simulink model "nms_model"  (R2020a)
settings: Solver=ode15s  StartTime=0.0  StopTime=2.6  MaxStep=.01  RelTol=1e-4  AbsTol=1e-6  EnableMultiTasking=on
values from neighbouring files (symbols this model uses):
  dt_visual = -1    [NMScontrol.m]    (also in runmodel.m = 0.001)
  g = params.g    [NMPCcostFunction.m]    (also in dynamicsNMPC.m = 9.81)
  m = parametersOpt(1)    [CGBgreybox.m]    (also in NMPCcostFunction.m = params.m)
undefined symbols (not defined in the file or in its folder): hatLeftHipToCenterDistWidth, initialTargetAngle, LongDelay, LongLoopDelay, LPreStimBFSHinit, LPreStimGASinit, LPreStimGLUinit, LPreStimHABinit, LPreStimHADinit, LPreStimHAMinit, LPreStimHFLinit, LPreStimRFinit, LPreStimSOLinit, LPreStimTAinit, LPreStimVASinit, LTargetAngleInit, LTargetAngleRInit, MidDelay, RPreStimBFSHinit, RPreStimGASinit, RPreStimGLUinit, RPreStimHABinit, RPreStimHADinit, RPreStimHAMinit, RPreStimHFLinit, RPreStimRFinit, RPreStimSOLinit, RPreStimTAinit, RPreStimVASinit, RTargetAngleInit, RTargetAngleRInit, ShortDelay, termination_height, thetaHATref, X, Y, Z
libraries: NeuroMuscularLibrary x107, nesl_utility x25, sm_lib x16, simulink x3
(part 3 of 3)

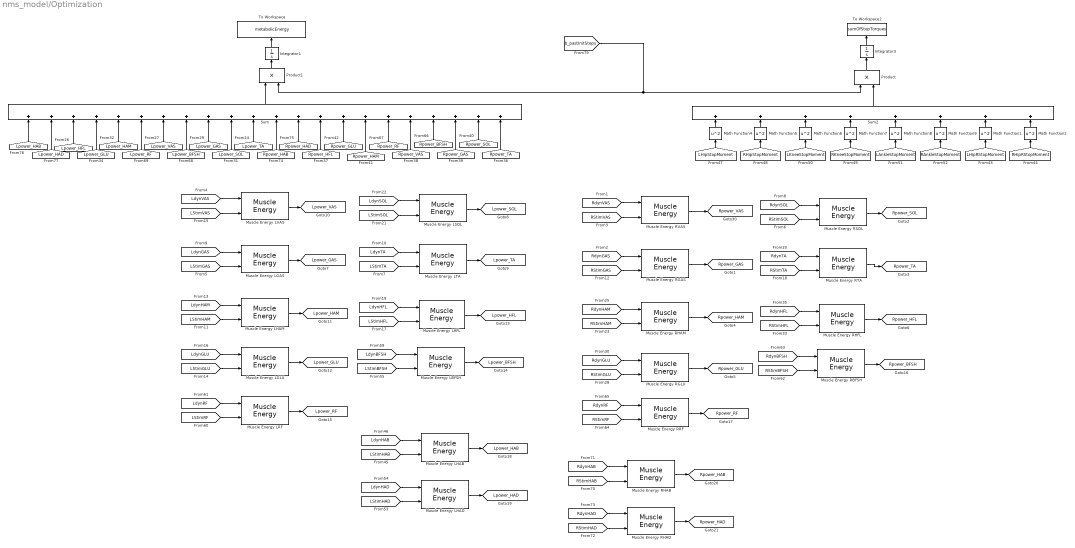
== system nms_model/Optimization ==
  Integrator1 : Integrator
  Integrator3 : Integrator
  Math Function{1..2,4..9} (8 alike) : Math  Operator=square  SignedPower=on  SaturateOnIntegerOverflow=on
  Muscle Energy LBFSH : NeuroMuscularLibrary/Muscle Energy  lopt=loptBFSH  FT=FT_BFSH  Fmax=FmaxBFSH  vmax=vmaxBFSH
  Muscle Energy LGAS : NeuroMuscularLibrary/Muscle Energy  lopt=loptGAS  FT=FT_GAS  Fmax=FmaxGAS  vmax=vmaxGAS
  Muscle Energy LGLU : NeuroMuscularLibrary/Muscle Energy  lopt=loptGLU  FT=FT_GLU  Fmax=FmaxGLU  vmax=vmaxGLU
  Muscle Energy LHAB : NeuroMuscularLibrary/Muscle Energy  lopt=loptHAB  FT=FT_HAB  Fmax=FmaxHAB  vmax=vmaxHAB
  Muscle Energy LHAD : NeuroMuscularLibrary/Muscle Energy  lopt=loptHAD  FT=FT_HAD  Fmax=FmaxHAD  vmax=vmaxHAD
  Muscle Energy LHAM : NeuroMuscularLibrary/Muscle Energy  lopt=loptHAM  FT=FT_HAM  Fmax=FmaxHAM  vmax=vmaxHAM
  Muscle Energy LHFL : NeuroMuscularLibrary/Muscle Energy  lopt=loptHFL  FT=FT_HFL  Fmax=FmaxHFL  vmax=vmaxHFL
  Muscle Energy LRF : NeuroMuscularLibrary/Muscle Energy  lopt=loptRF  FT=FT_RF  Fmax=FmaxRF  vmax=vmaxRF
  Muscle Energy LSOL : NeuroMuscularLibrary/Muscle Energy  lopt=loptSOL  FT=FT_SOL  Fmax=FmaxSOL  vmax=vmaxSOL
  Muscle Energy LTA : NeuroMuscularLibrary/Muscle Energy  lopt=loptTA  FT=FT_TA  Fmax=FmaxTA  vmax=vmaxTA
  Muscle Energy LVAS : NeuroMuscularLibrary/Muscle Energy  lopt=loptVAS  FT=FT_VAS  Fmax=FmaxVAS  vmax=vmaxVAS
  Muscle Energy RBFSH : NeuroMuscularLibrary/Muscle Energy  lopt=loptBFSH  FT=FT_BFSH  Fmax=FmaxBFSH  vmax=vmaxBFSH
  Muscle Energy RGAS : NeuroMuscularLibrary/Muscle Energy  lopt=loptGAS  FT=FT_GAS  Fmax=FmaxGAS  vmax=vmaxGAS
  Muscle Energy RGLU : NeuroMuscularLibrary/Muscle Energy  lopt=loptGLU  FT=FT_GLU  Fmax=FmaxGLU  vmax=vmaxGLU
  Muscle Energy RHAB : NeuroMuscularLibrary/Muscle Energy  lopt=loptHAB  FT=FT_HAB  Fmax=FmaxHAB  vmax=vmaxHAB
  Muscle Energy RHAD : NeuroMuscularLibrary/Muscle Energy  lopt=loptHAD  FT=FT_HAD  Fmax=FmaxHAD  vmax=vmaxHAD
  Muscle Energy RHAM : NeuroMuscularLibrary/Muscle Energy  lopt=loptHAM  FT=FT_HAM  Fmax=FmaxHAM  vmax=vmaxHAM
  Muscle Energy RHFL : NeuroMuscularLibrary/Muscle Energy  lopt=loptHFL  FT=FT_HFL  Fmax=FmaxHFL  vmax=vmaxHFL
  Muscle Energy RRF : NeuroMuscularLibrary/Muscle Energy  lopt=loptRF  FT=FT_RF  Fmax=FmaxRF  vmax=vmaxRF
  Muscle Energy RSOL : NeuroMuscularLibrary/Muscle Energy  lopt=loptSOL  FT=FT_SOL  Fmax=FmaxSOL  vmax=vmaxSOL
  Muscle Energy RTA : NeuroMuscularLibrary/Muscle Energy  lopt=loptTA  FT=FT_TA  Fmax=FmaxTA  vmax=vmaxTA
  Muscle Energy RVAS : NeuroMuscularLibrary/Muscle Energy  lopt=loptVAS  FT=FT_VAS  Fmax=FmaxVAS  vmax=vmaxVAS
  Product : Product
  Product1 : Product
  Sum : Sum  Inputs=++++++++++++++++++++++
  Sum2 : Sum  Inputs=++++++++
  To Workspace : ToWorkspace  VariableName=metabolicEnergy  SampleTime=-1
      settings: MaxDataPoints=1
  To Workspace2 : ToWorkspace  VariableName=sumOfStopTorques  SampleTime=-1
      settings: MaxDataPoints=1
  tag scope: Lpower_BFSH=global, Lpower_GAS=global, Lpower_GLU=global, Lpower_HAB=global, Lpower_HAD=global, Lpower_HAM=global, Lpower_HFL=global, Lpower_RF=global, Lpower_SOL=global, Lpower_TA=global, Lpower_VAS=global, Rpower_BFSH=global, Rpower_GAS=global, Rpower_GLU=global, Rpower_HAB=global, Rpower_HAD=global, Rpower_HAM=global, Rpower_HFL=global, Rpower_RF=global, Rpower_SOL=global, Rpower_TA=global, Rpower_VAS=global
  wires:
  [RdynSOL] -> Muscle Energy RSOL/1
  [RStimSOL] -> Muscle Energy RSOL/2
  [RStimVAS] -> Muscle Energy RVAS/2
  [RStimGAS] -> Muscle Energy RGAS/2
  Muscle Energy RVAS/1 -> [Rpower_VAS]
  Muscle Energy RGAS/1 -> [Rpower_GAS]
  Muscle Energy RSOL/1 -> [Rpower_SOL]
  Muscle Energy RTA/1 -> [Rpower_TA]
  [RdynTA] -> Muscle Energy RTA/1
  [RStimTA] -> Muscle Energy RTA/2
  [RdynHAM] -> Muscle Energy RHAM/1
  [RStimHAM] -> Muscle Energy RHAM/2
  [RdynGLU] -> Muscle Energy RGLU/1
  [RStimGLU] -> Muscle Energy RGLU/2
  [RdynHFL] -> Muscle Energy RHFL/1
  [RStimHFL] -> Muscle Energy RHFL/2
  Muscle Energy RHAM/1 -> [Rpower_HAM]
  Muscle Energy RGLU/1 -> [Rpower_GLU]
  Muscle Energy RHFL/1 -> [Rpower_HFL]
  [Lpower_HAB] -> Sum/1
  [Lpower_VAS] -> Sum/7
  [Lpower_RF] -> Sum/6
  [Lpower_HAM] -> Sum/5
  [Lpower_GLU] -> Sum/4
  [Lpower_HFL] -> Sum/3
  [Lpower_HAD] -> Sum/2
  [RdynGAS] -> Muscle Energy RGAS/1
  [RdynVAS] -> Muscle Energy RVAS/1
  [LdynSOL] -> Muscle Energy LSOL/1
  [LStimSOL] -> Muscle Energy LSOL/2
  [LStimVAS] -> Muscle Energy LVAS/2
  [LStimGAS] -> Muscle Energy LGAS/2
  Muscle Energy LVAS/1 -> [Lpower_VAS]
  Muscle Energy LGAS/1 -> [Lpower_GAS]
  Muscle Energy LSOL/1 -> [Lpower_SOL]
  Muscle Energy LTA/1 -> [Lpower_TA]
  [LdynTA] -> Muscle Energy LTA/1
  [LStimTA] -> Muscle Energy LTA/2
  [LdynHAM] -> Muscle Energy LHAM/1
  [LStimHAM] -> Muscle Energy LHAM/2
  [LdynGLU] -> Muscle Energy LGLU/1
  [LStimGLU] -> Muscle Energy LGLU/2
  [LdynHFL] -> Muscle Energy LHFL/1
  [LStimHFL] -> Muscle Energy LHFL/2
  Muscle Energy LHAM/1 -> [Lpower_HAM]
  Muscle Energy LGLU/1 -> [Lpower_GLU]
  Muscle Energy LHFL/1 -> [Lpower_HFL]
  [LdynGAS] -> Muscle Energy LGAS/1
  [LdynVAS] -> Muscle Energy LVAS/1
  [Lpower_SOL] -> Sum/10
  [Rpower_HAM] -> Sum/16
  [Rpower_GLU] -> Sum/15
  [Rpower_HFL] -> Sum/14
  [Rpower_HAD] -> Sum/13
  [Rpower_HAB] -> Sum/12
  [Lpower_TA] -> Sum/11
  Integrator1/1 -> To Workspace/1
  Sum/1 -> Product1/1
  Integrator3/1 -> To Workspace2/1
  Math Function4/1 -> Sum2/1
  [LHipStopMoment] -> Math Function4/1
  Math Function5/1 -> Sum2/2
  [RHipStopMoment] -> Math Function5/1
  Math Function6/1 -> Sum2/3
  Math Function7/1 -> Sum2/4
  [LKneeStopMoment] -> Math Function6/1
  [RKneeStopMoment] -> Math Function7/1
  [LAnkleStopMoment] -> Math Function8/1
  Math Function8/1 -> Sum2/5
  [RAnkleStopMoment] -> Math Function9/1
  Math Function9/1 -> Sum2/6
  Product/1 -> Integrator3/1
  Sum2/1 -> Product/2
  Product1/1 -> Integrator1/1
  Muscle Energy LBFSH/1 -> [Lpower_BFSH]
  [LStimBFSH] -> Muscle Energy LBFSH/2
  [LdynBFSH] -> Muscle Energy LBFSH/1
  [LdynRF] -> Muscle Energy LRF/1
  [LStimRF] -> Muscle Energy LRF/2
  Muscle Energy LRF/1 -> [Lpower_RF]
  Muscle Energy RRF/1 -> [Rpower_RF]
  [RdynRF] -> Muscle Energy RRF/1
  Muscle Energy RBFSH/1 -> [Rpower_BFSH]
  [RStimRF] -> Muscle Energy RRF/2
  [RStimBFSH] -> Muscle Energy RBFSH/2
  [RdynBFSH] -> Muscle Energy RBFSH/1
  [Lpower_BFSH] -> Sum/8
  [Lpower_GAS] -> Sum/9
  [Rpower_VAS] -> Sum/18
  [Rpower_RF] -> Sum/17
  Math Function1/1 -> Sum2/7
  [LHipRStopMoment] -> Math Function1/1
  [RHipRStopMoment] -> Math Function2/1
  Muscle Energy LHAB/1 -> [Lpower_HAB]
  [LStimHAB] -> Muscle Energy LHAB/2
  [LdynHAB] -> Muscle Energy LHAB/1
  [LdynHAD] -> Muscle Energy LHAD/1
  [LStimHAD] -> Muscle Energy LHAD/2
  Muscle Energy LHAD/1 -> [Lpower_HAD]
  Muscle Energy RHAD/1 -> [Rpower_HAD]
  [RStimHAD] -> Muscle Energy RHAD/2
  [RdynHAD] -> Muscle Energy RHAD/1
  [RdynHAB] -> Muscle Energy RHAB/1
  [RStimHAB] -> Muscle Energy RHAB/2
  Muscle Energy RHAB/1 -> [Rpower_HAB]
  [Rpower_TA] -> Sum/22
  [Rpower_SOL] -> Sum/21
  [Rpower_GAS] -> Sum/20
  [Rpower_BFSH] -> Sum/19
  Math Function2/1 -> Sum2/8
  [b_pastInitSteps] -> Product/1, Product1/2

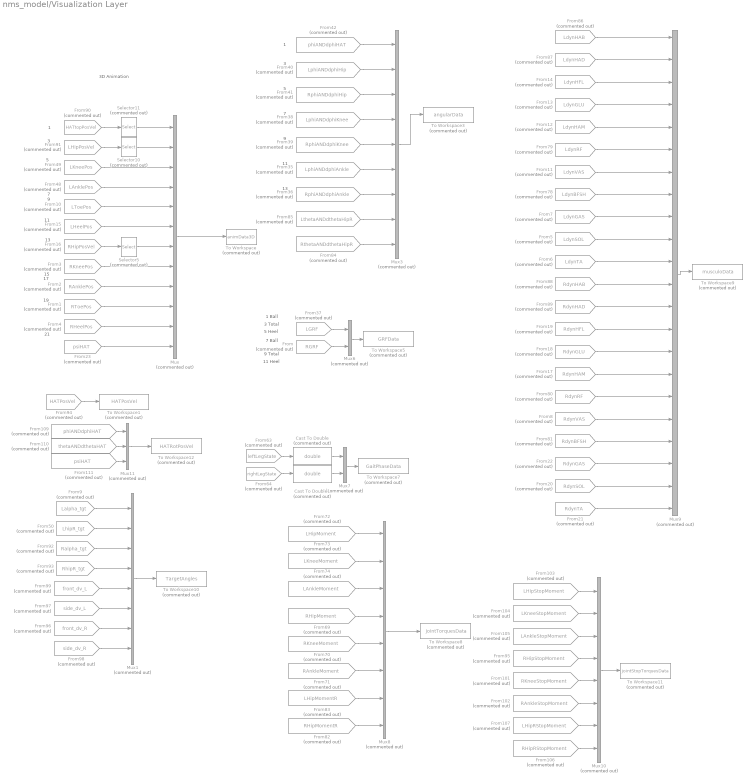
== system nms_model/Visualization Layer ==
  note: 21
  note: 19
  note: 17
  note: 15
  note: 13
  note: 11
  note: 9
  note: 7
  note: 5
  note: 3
  note: 1
  note: 3D Animation
  note: 1
  note: 13
  note: 3
  note: 5
  note: 7
  note: 9
  note: 11
  note: 9 Total
  note: 1 Ball
  note: 5 Heel
  note: 11 Heel
  note: 3 Total
  note: 7 Ball
  Cast To Double : DataTypeConversion  Commented=on  OutDataTypeStr=double
  Cast To Double1 : DataTypeConversion  Commented=on  OutDataTypeStr=double
  From : From  Commented=on  GotoTag=RGRF  TagVisibility=global
  From1 : From  Commented=on  GotoTag=RToePos  TagVisibility=global
      settings: CloseFcn=tagdialog Close
  From10 : From  Commented=on  GotoTag=LToePos  TagVisibility=global
      settings: CloseFcn=tagdialog Close
  From101 : From  Commented=on  GotoTag=RKneeStopMoment  TagVisibility=global
  From102 : From  Commented=on  GotoTag=RAnkleStopMoment  TagVisibility=global
  From103 : From  Commented=on  GotoTag=LHipStopMoment  TagVisibility=global
  From104 : From  Commented=on  GotoTag=LKneeStopMoment  TagVisibility=global
  From105 : From  Commented=on  GotoTag=LAnkleStopMoment  TagVisibility=global
  From106 : From  Commented=on  GotoTag=RHipRStopMoment  TagVisibility=global
  From107 : From  Commented=on  GotoTag=LHipRStopMoment  TagVisibility=global
  From109 : From  Commented=on  GotoTag=phiANDdphiHAT  TagVisibility=global
  From11 : From  Commented=on  GotoTag=LdynVAS  TagVisibility=global
  From110 : From  Commented=on  GotoTag=thetaANDdthetaHAT  TagVisibility=global
  From111 : From  Commented=on  GotoTag=psiHAT  TagVisibility=global
  From12 : From  Commented=on  GotoTag=LdynHAM  TagVisibility=global
  From13 : From  Commented=on  GotoTag=LdynGLU  TagVisibility=global
  From14 : From  Commented=on  GotoTag=LdynHFL  TagVisibility=global
  From15 : From  Commented=on  GotoTag=LHeelPos  TagVisibility=global
      settings: CloseFcn=tagdialog Close
  From16 : From  Commented=on  GotoTag=RHipPosVel  TagVisibility=global
  From17 : From  Commented=on  GotoTag=RdynHAM  TagVisibility=global
  From18 : From  Commented=on  GotoTag=RdynGLU  TagVisibility=global
  From19 : From  Commented=on  GotoTag=RdynHFL  TagVisibility=global
  From2 : From  Commented=on  GotoTag=RAnklePos  TagVisibility=global
      settings: CloseFcn=tagdialog Close
  From20 : From  Commented=on  GotoTag=RdynSOL  TagVisibility=global
  From21 : From  Commented=on  GotoTag=RdynTA  TagVisibility=global
  From22 : From  Commented=on  GotoTag=RdynGAS  TagVisibility=global
  From23 : From  Commented=on  GotoTag=psiHAT  TagVisibility=global
  From3 : From  Commented=on  GotoTag=RKneePos  TagVisibility=global
      settings: CloseFcn=tagdialog Close
  From35 : From  Commented=on  GotoTag=LphiANDdphiAnkle  TagVisibility=global
  From36 : From  Commented=on  GotoTag=RphiANDdphiAnkle  TagVisibility=global
  From37 : From  Commented=on  GotoTag=LGRF  TagVisibility=global
  From38 : From  Commented=on  GotoTag=LphiANDdphiKnee  TagVisibility=global
  From39 : From  Commented=on  GotoTag=RphiANDdphiKnee  TagVisibility=global
  From4 : From  Commented=on  GotoTag=RHeelPos  TagVisibility=global
      settings: CloseFcn=tagdialog Close
  From40 : From  Commented=on  GotoTag=LphiANDdphiHip  TagVisibility=global
  From41 : From  Commented=on  GotoTag=RphiANDdphiHip  TagVisibility=global
  From42 : From  Commented=on  GotoTag=phiANDdphiHAT  TagVisibility=global
  From48 : From  Commented=on  GotoTag=LAnklePos  TagVisibility=global
      settings: CloseFcn=tagdialog Close
  From49 : From  Commented=on  GotoTag=LKneePos  TagVisibility=global
      settings: CloseFcn=tagdialog Close
  From5 : From  Commented=on  GotoTag=LdynSOL  TagVisibility=global
  From50 : From  Commented=on  GotoTag=LhipR_tgt  TagVisibility=global
  From6 : From  Commented=on  GotoTag=LdynTA  TagVisibility=global
  From63 : From  Commented=on  GotoTag=leftLegState  TagVisibility=global
  From64 : From  Commented=on  GotoTag=rightLegState  TagVisibility=global
  From69 : From  Commented=on  GotoTag=RHipMoment  TagVisibility=global
  From7 : From  Commented=on  GotoTag=LdynGAS  TagVisibility=global
  From70 : From  Commented=on  GotoTag=RKneeMoment  TagVisibility=global
  From71 : From  Commented=on  GotoTag=RAnkleMoment  TagVisibility=global
  From72 : From  Commented=on  GotoTag=LHipMoment  TagVisibility=global
  From73 : From  Commented=on  GotoTag=LKneeMoment  TagVisibility=global
  From74 : From  Commented=on  GotoTag=LAnkleMoment  TagVisibility=global
  From78 : From  Commented=on  GotoTag=LdynBFSH  TagVisibility=global
  From79 : From  Commented=on  GotoTag=LdynRF  TagVisibility=global
  From8 : From  Commented=on  GotoTag=RdynVAS  TagVisibility=global
  From80 : From  Commented=on  GotoTag=RdynRF  TagVisibility=global
  From81 : From  Commented=on  GotoTag=RdynBFSH  TagVisibility=global
  From82 : From  Commented=on  GotoTag=RHipMomentR  TagVisibility=global
  From83 : From  Commented=on  GotoTag=LHipMomentR  TagVisibility=global
  From84 : From  Commented=on  GotoTag=RthetaANDdthetaHipR  TagVisibility=global
  From85 : From  Commented=on  GotoTag=LthetaANDdthetaHipR  TagVisibility=global
  From86 : From  Commented=on  GotoTag=LdynHAB  TagVisibility=global
  From87 : From  Commented=on  GotoTag=LdynHAD  TagVisibility=global
  From88 : From  Commented=on  GotoTag=RdynHAB  TagVisibility=global
  From89 : From  Commented=on  GotoTag=RdynHAD  TagVisibility=global
  From9 : From  Commented=on  GotoTag=Lalpha_tgt  TagVisibility=global
  From90 : From  Commented=on  GotoTag=HATtopPosVel  TagVisibility=global
  From91 : From  Commented=on  GotoTag=LHipPosVel  TagVisibility=global
  From92 : From  Commented=on  GotoTag=Ralpha_tgt  TagVisibility=global
  From93 : From  Commented=on  GotoTag=RhipR_tgt  TagVisibility=global
  From94 : From  Commented=on  GotoTag=HATPosVel  TagVisibility=global
  From95 : From  Commented=on  GotoTag=RHipStopMoment  TagVisibility=global
  From96 : From  Commented=on  GotoTag=front_dv_R  TagVisibility=global
      settings: CloseFcn=tagdialog Close
  From97 : From  Commented=on  GotoTag=side_dv_L  TagVisibility=global
      settings: CloseFcn=tagdialog Close
  From98 : From  Commented=on  GotoTag=side_dv_R  TagVisibility=global
      settings: CloseFcn=tagdialog Close
  From99 : From  Commented=on  GotoTag=front_dv_L  TagVisibility=global
      settings: CloseFcn=tagdialog Close
  Mux : Mux  Commented=on  Inputs=12
  Mux1 : Mux  Commented=on  Inputs=8
  Mux10 : Mux  Commented=on  Inputs=8
  Mux11 : Mux  Commented=on  Inputs=3
  Mux3 : Mux  Commented=on  Inputs=9
  Mux6 : Mux  Commented=on  Inputs=2
  Mux7 : Mux  Commented=on  Inputs=2
  Mux8 : Mux  Commented=on  Inputs=8
  Mux9 : Mux  Commented=on  Inputs=22
  Selector10 : Selector  Commented=on  InputPortWidth=6  IndexOptions=Index vector (dialog)  Indices=[1 2 3]  OutputSizes=1
  Selector11 : Selector  Commented=on  InputPortWidth=6  IndexOptions=Index vector (dialog)  Indices=[1 2 3]  OutputSizes=1
  Selector5 : Selector  Commented=on  InputPortWidth=6  IndexOptions=Index vector (dialog)  Indices=[1 2 3]  OutputSizes=1
  To Workspace : ToWorkspace  Commented=on  VariableName=animData3D  SaveFormat=Structure With Time  SampleTime=-1
  To Workspace1 : ToWorkspace  Commented=on  VariableName=HATPosVel  SaveFormat=Structure With Time  SampleTime=dt_visual
  To Workspace10 : ToWorkspace  Commented=on  VariableName=TargetAngles  SaveFormat=Structure With Time  SampleTime=dt_visual
  To Workspace11 : ToWorkspace  Commented=on  VariableName=jointStopTorquesData  SaveFormat=Structure With Time  SampleTime=dt_visual
  To Workspace12 : ToWorkspace  Commented=on  VariableName=HATRotPosVel  SaveFormat=Structure With Time  SampleTime=dt_visual
  To Workspace3 : ToWorkspace  Commented=on  VariableName=angularData  SaveFormat=Structure With Time  SampleTime=dt_visual
  To Workspace5 : ToWorkspace  Commented=on  VariableName=GRFData  SaveFormat=Structure With Time  SampleTime=dt_visual
  To Workspace7 : ToWorkspace  Commented=on  VariableName=GaitPhaseData  SaveFormat=Structure With Time  SampleTime=dt_visual
  To Workspace8 : ToWorkspace  Commented=on  VariableName=jointTorquesData  SaveFormat=Structure With Time  SampleTime=dt_visual
  To Workspace9 : ToWorkspace  Commented=on  VariableName=musculoData  SaveFormat=Structure With Time  SampleTime=dt_visual
  wires:
  From16/1 -> Selector5/1
  From90/1 -> Selector11/1
  From91/1 -> Selector10/1
  Selector11/1 -> Mux/1
  From2/1 -> Mux/9
  From3/1 -> Mux/8
  Selector5/1 -> Mux/7
  From15/1 -> Mux/6
  From10/1 -> Mux/5
  From48/1 -> Mux/4
  From49/1 -> Mux/3
  Selector10/1 -> Mux/2
  Mux/1 -> To Workspace/1
  From4/1 -> Mux/11
  From1/1 -> Mux/10
  From36/1 -> Mux3/7
  Mux6/1 -> To Workspace5/1
  From/1 -> Mux6/2
  From42/1 -> Mux3/1
  Mux3/1 -> To Workspace3/1
  From35/1 -> Mux3/6
  From38/1 -> Mux3/4
  From37/1 -> Mux6/1
  From40/1 -> Mux3/2
  From39/1 -> Mux3/5
  From41/1 -> Mux3/3
  From64/1 -> Cast To Double1/1
  Mux7/1 -> To Workspace7/1
  From63/1 -> Cast To Double/1
  Mux8/1 -> To Workspace8/1
  From72/1 -> Mux8/1
  From73/1 -> Mux8/2
  From74/1 -> Mux8/3
  From69/1 -> Mux8/4
  From70/1 -> Mux8/5
  From71/1 -> Mux8/6
  Mux9/1 -> To Workspace9/1
  From17/1 -> Mux9/16
  From14/1 -> Mux9/3
  From18/1 -> Mux9/15
  From8/1 -> Mux9/18
  From78/1 -> Mux9/8
  From22/1 -> Mux9/20
  From81/1 -> Mux9/19
  From11/1 -> Mux9/7
  From7/1 -> Mux9/9
  From5/1 -> Mux9/10
  From79/1 -> Mux9/6
  From12/1 -> Mux9/5
  From13/1 -> Mux9/4
  From6/1 -> Mux9/11
  From80/1 -> Mux9/17
  From19/1 -> Mux9/14
  From20/1 -> Mux9/21
  From21/1 -> Mux9/22
  From83/1 -> Mux8/7
  From82/1 -> Mux8/8
  From85/1 -> Mux3/8
  From84/1 -> Mux3/9
  From88/1 -> Mux9/12
  From89/1 -> Mux9/13
  From86/1 -> Mux9/1
  From87/1 -> Mux9/2
  From94/1 -> To Workspace1/1
  From99/1 -> Mux1/5
  From92/1 -> Mux1/3
  From93/1 -> Mux1/4
  Mux1/1 -> To Workspace10/1
  From96/1 -> Mux1/7
  From50/1 -> Mux1/2
  From98/1 -> Mux1/8
  From97/1 -> Mux1/6
  From9/1 -> Mux1/1
  From102/1 -> Mux10/6
  From95/1 -> Mux10/4
  From104/1 -> Mux10/2
  Mux10/1 -> To Workspace11/1
  From103/1 -> Mux10/1
  From101/1 -> Mux10/5
  From105/1 -> Mux10/3
  From107/1 -> Mux10/7
  From106/1 -> Mux10/8
  Mux11/1 -> To Workspace12/1
  From110/1 -> Mux11/2
  From111/1 -> Mux11/3
  From109/1 -> Mux11/1
  From23/1 -> Mux/12
  Cast To Double/1 -> Mux7/1
  Cast To Double1/1 -> Mux7/2

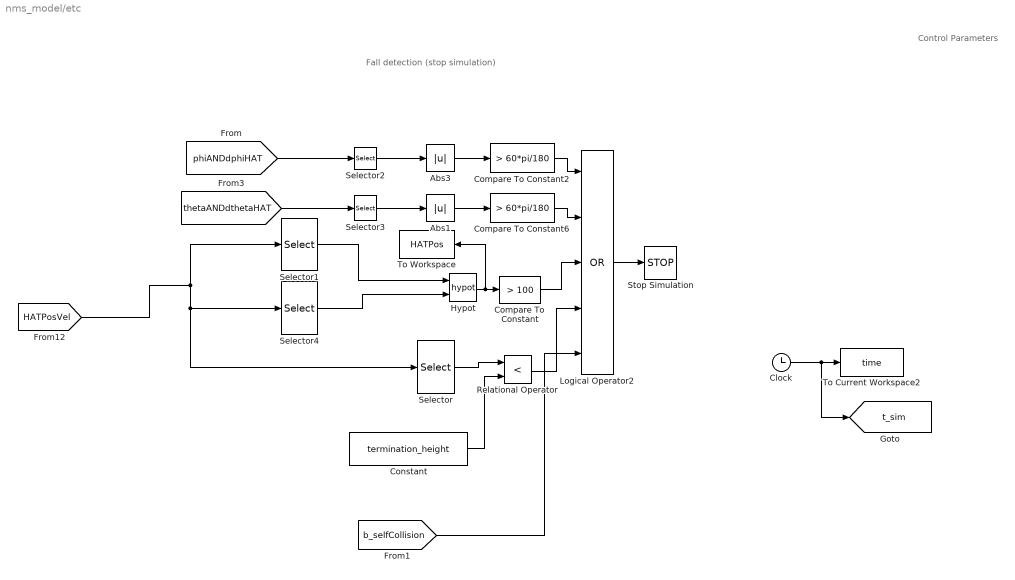
== system nms_model/etc ==
  note: Fall detection
      | (stop simulation)
  note: Control Parameters
  Abs1 : Abs
  Abs3 : Abs
  Clock : Clock
  Compare To Constant : simulink/Logic and Bit Operations/Compare To Constant  relop=>  const=100  OutDataTypeStr=boolean
  Compare To Constant2 : simulink/Logic and Bit Operations/Compare To Constant  relop=>  const=60*pi/180  OutDataTypeStr=boolean
  Compare To Constant6 : simulink/Logic and Bit Operations/Compare To Constant  relop=>  const=60*pi/180  OutDataTypeStr=boolean
  Constant : Constant  Value=termination_height
  Hypot : Math  Operator=hypot  SaturateOnIntegerOverflow=on
  Logical Operator2 : Logic  Operator=OR  Inputs=5  AllPortsSameDT=off  OutDataTypeStr=boolean
  Relational Operator : RelationalOperator  Operator=<  OutDataTypeStr=boolean  RndMeth=Nearest
  Selector : Selector  InputPortWidth=6  IndexOptions=Index vector (dialog)  Indices=[3]  OutputSizes=1
  Selector1 : Selector  InputPortWidth=6  IndexOptions=Index vector (dialog)  Indices=[1]  OutputSizes=1
  Selector2 : Selector  InputPortWidth=2  IndexOptions=Index vector (dialog)  Indices=[1]  OutputSizes=1
  Selector3 : Selector  InputPortWidth=2  IndexOptions=Index vector (dialog)  Indices=[1]  OutputSizes=1
  Selector4 : Selector  InputPortWidth=6  IndexOptions=Index vector (dialog)  Indices=[2]  OutputSizes=1
  Stop Simulation : Stop
  To Current Workspace2 : ToWorkspace  VariableName=time  SampleTime=-1
      settings: MaxDataPoints=1
  To Workspace : ToWorkspace  VariableName=HATPos  SampleTime=-1
      settings: MaxDataPoints=1
  tag scope: t_sim=global
  wires:
  Selector2/1 -> Abs3/1
  Abs3/1 -> Compare To Constant2/1
  Compare To Constant2/1 -> Logical Operator2/1
  Logical Operator2/1 -> Stop Simulation/1
  Selector3/1 -> Abs1/1
  Abs1/1 -> Compare To Constant6/1
  Compare To Constant6/1 -> Logical Operator2/2
  Compare To Constant/1 -> Logical Operator2/3
  Selector/1 -> Relational Operator/1
  Selector1/1 -> Hypot/1
  Constant/1 -> Relational Operator/2
  Relational Operator/1 -> Logical Operator2/4
  [HATPosVel] -> Selector1/1, Selector/1, Selector4/1
  Clock/1 -> [t_sim], To Current Workspace2/1
  [phiANDdphiHAT] -> Selector2/1
  [thetaANDdthetaHAT] -> Selector3/1
  Selector4/1 -> Hypot/2
  Hypot/1 -> To Workspace/1, Compare To Constant/1
  [b_selfCollision] -> Logical Operator2/5

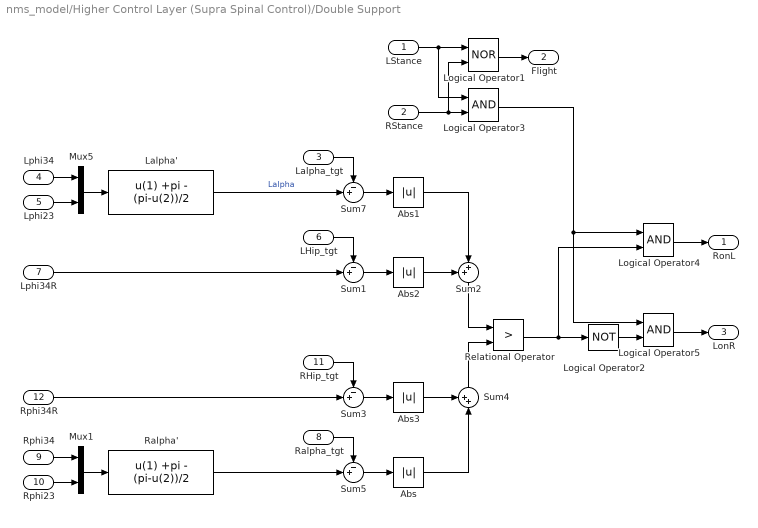
== system nms_model/Higher Control Layer (Supra Spinal Control)/Double Support ==
  LStance : Inport
  RStance : Inport  Port=2
  Lalpha_tgt : Inport  Port=3
  Lphi34 : Inport  Port=4
  Lphi23 : Inport  Port=5
  LHip_tgt : Inport  Port=6
  Lphi34R : Inport  Port=7
  Ralpha_tgt : Inport  Port=8
  Rphi34 : Inport  Port=9
  Rphi23 : Inport  Port=10
  RHip_tgt : Inport  Port=11
  Rphi34R : Inport  Port=12
  Abs{,1..3} (4 alike) : Abs  ZeroCross=off
  Lalpha' : Fcn  Expr=u(1) +pi - (pi-u(2))/2
  Logical Operator1 : Logic  Operator=NOR  AllPortsSameDT=off  OutDataTypeStr=boolean
  Logical Operator2 : Logic  Operator=NOT  AllPortsSameDT=off
  Logical Operator3 : Logic  AllPortsSameDT=off
  Logical Operator4 : Logic  AllPortsSameDT=off
  Logical Operator5 : Logic  AllPortsSameDT=off
  Mux1 : Mux  Inputs=2
  Mux5 : Mux  Inputs=2
  Ralpha' : Fcn  Expr=u(1) +pi - (pi-u(2))/2
  Relational Operator : RelationalOperator  Operator=>  ZeroCross=off  RndMeth=Nearest
  Sum{1,3,5,7} (4 alike) : Sum  Inputs=-+|
  Sum2 : Sum  Inputs=++|
  Sum4 : Sum  Inputs=++|
  RonL : Outport
  Flight : Outport  Port=2
  LonR : Outport  Port=3
  wires:
  Lalpha'/1 -> Sum7/2  "Lalpha"
  Mux5/1 -> Lalpha'/1
  Ralpha'/1 -> Sum5/2
  Mux1/1 -> Ralpha'/1
  Sum5/1 -> Abs/1
  Sum7/1 -> Abs1/1
  LStance/1 -> Logical Operator3/1, Logical Operator1/1
  RStance/1 -> Logical Operator3/2, Logical Operator1/2
  Lalpha_tgt/1 -> Sum7/1
  Lphi34/1 -> Mux5/1
  Lphi23/1 -> Mux5/2
  Ralpha_tgt/1 -> Sum5/1
  Rphi34/1 -> Mux1/1
  Rphi23/1 -> Mux1/2
  Logical Operator1/1 -> Flight/1
  LHip_tgt/1 -> Sum1/1
  Lphi34R/1 -> Sum1/2
  Sum1/1 -> Abs2/1
  Abs2/1 -> Sum2/1
  Abs1/1 -> Sum2/2
  Sum2/1 -> Relational Operator/1
  RHip_tgt/1 -> Sum3/1
  Rphi34R/1 -> Sum3/2
  Sum3/1 -> Abs3/1
  Abs/1 -> Sum4/2
  Abs3/1 -> Sum4/1
  Sum4/1 -> Relational Operator/2
  Logical Operator4/1 -> RonL/1
  Logical Operator2/1 -> Logical Operator5/2
  Logical Operator5/1 -> LonR/1
  Relational Operator/1 -> Logical Operator2/1, Logical Operator4/2
  Logical Operator3/1 -> Logical Operator5/1, Logical Operator4/1
